simulink model "fuzzy"  (R2018b)
settings: Solver=VariableStepAuto  StartTime=0.0  StopTime=10.0  RelTol=1e-3
libraries: fuzblock x1, simulink_extras x1
settings Model: Creator=student  LastModifiedBy=student

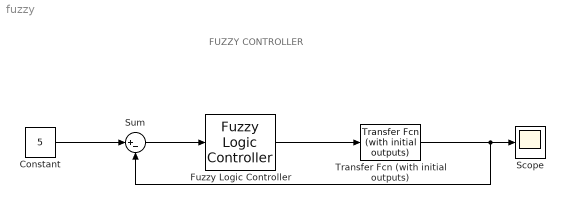
== system fuzzy ==
  note: FUZZY CONTROLLER
  Constant : Constant  Value=5
  Fuzzy Logic Controller : fuzblock/Fuzzy Logic  Controller  FIS='fuzzycontroller.fis'  OutputSampleNumber=101  DataType=double  FuzzifiedInputs=off  RuleFiringStrengths=off  RuleOutputs=off  AggregatedOutputs=off  SimulateUsing=Interpreted execution  OutOfRangeInputValueMessage=warning  NoRuleFiredMessage=warning  EmptyOutputFuzzySetMessage=warning
  Scope : Scope
  Sum : Sum  Inputs=|+-
  Transfer Fcn (with initial outputs) : simulink_extras/Additional Linear/Transfer Fcn (with initial outputs)  N=[1]  D="[1  5]"  Y0=.5  U0=0
  wires:
  Fuzzy Logic Controller/1 -> Transfer Fcn (with initial outputs)/1
  Constant/1 -> Sum/1
  Sum/1 -> Fuzzy Logic Controller/1
  Transfer Fcn (with initial outputs)/1 -> Sum/2, Scope/1
